simulink model "model"  (R2020b)
settings: Solver=VariableStepAuto  StartTime=0.0  StopTime=settings.Tsim  FixedStep=0.1  RelTol=1e-6  AbsTol=1e-6
values from neighbouring files (symbols this model uses):
  D = date(3)    [date2jd.m]
  settings = Simulink.Parameter    [main.m]
libraries: vrlib x10
(part 2 of 2)

== matlab function model/disturbanceTorques ==
  data: J input; M_disturbance output; r_CG input; A_BN input; A_BL input; S_B input; rr input; vv input; C_D input; rho input; t input; b_B output
function [M_disturbance, b_B] = disturbanceTorquesa(J, r_CG, A_BN, A_BL, S_B, rr, vv, C_D, rho, t)



G = 6.67408e-11;
m_E = 5.972e+24;
kep = car2par(rr, vv, 398600);
a = kep(1); e = kep(2); i = kep(3);
OM = kep(4); om = kep(5); th = kep(6);
R_equat = 6371e+3; % [m]
p = a*(1-e^2);
R = p / (1+e*cos(th)) * 1e+3; % [m]





% Moments of Inertia [kg*m^2]
% (12U Cubesat)
J1 = J(1,1);
J2 = J(2,2);
J3 = J(3,3);





C1 = (J2-J3)/J1;
C2 = (J3-J1)/J2;
C3 = (J1-J2)/J3;






%% Gravity Gradient Torque
c = A_BL * [1;0;0];



M_GG = [- 3*G*m_E/R^3 *C1* c(3)*c(2);
- 3*G*m_E/R^3 *C2* c(1)*c(3);
- 3*G*m_E/R^3 *C3* c(2)*c(1)];



%% SRP Torque @ 600 Km (Direct Solar Rad. + Sun Rad. Reflected by Earth + Earth Rad.)
F_e = 1358 + 580 + 143.4; % [W/m^2]
P = F_e / (3*1e+8);



N_body = 6; % # main body surfaces
N_SP = 4; % # solar panel surfaces



U = 0.1; % 1U length



N = zeros(N_body+N_SP,3);
A = zeros(N_body+N_SP,1);
r = zeros(N_body+N_SP,3);
n1 = [1 0 0]; n2 = [0 1 0]; n3 = [0 0 1];
% S/C Main Body: Normals, Surface Coefficients, Areas
N(1,:) = n1; N(2,:) = n2; N(3,:) = n3;
N(4,:) = -n1; N(5,:) = -n2; N(6,:) = -n3;
rho_s_body = 0.6; rho_d_body = 0.1;
A(1:N_body) = [4 6 6 4 6 6]*U^2; % [m^2]



% Solar Panels: Normals, Surface Coefficients, Areas
N(7,:) = n1; N(8,:) = -n1; N(9,:) = n1; N(10,:) = -n1;
rho_s_SP = 0.6; rho_d_SP = 0.1;
A(N_body+1:N_body+N_SP) = [12 12 12 12]*U^2; % [m^2]



% L.u.c. a RF centered @ Geometric Center of S/C::
% we will use it to define the coordinates of each surface's center
% along w/ the coordinates of th CG w.r.t. GC
r(1,:) = [1.5 0 0]*U; r(2,:) = [0 1 0]*U; r(3,:) = [0 0 1]*U;
r(4,:) = [-1.5 0 0]*U; r(5,:) = [0 -1 0]*U; r(6,:) = [0 0 -1]*U;
r(7,:) = [0 5 0]*U; r(8,:) = [0 5 0]*U;
r(9,:) = [0 -5 0]*U; r(10,:) = [0 -5 0]*U;



S_B_norm = S_B / norm(S_B);



M_SRP = zeros(3,1);
for k = 1:N_body+N_SP
if k <= N_body
rho_s = rho_s_body; rho_d = rho_d_body;
else
rho_s = rho_s_SP; rho_d = rho_d_SP;
end



n_k = N(k,:)';
F_k = - P*A(k)*dot(S_B_norm,n_k) * ( (1-rho_s)*S_B_norm + (2*rho_s*dot(S_B_norm,n_k)+2/3*rho_d)*n_k );



if dot(S_B_norm, n_k) > 0
r_k = (r(k,:) - r_CG')';
M_SRP_k = cross(r_k, F_k);
else
M_SRP_k = zeros(3,1);
end



M_SRP = M_SRP + M_SRP_k;



end




%% Air-Drag Torque
w_E = 2*pi/(23*3600 + 56*60 + 4.09); % Earth's angular rate [rad/s]
mu_E = 398600.433; % [km^3/s^2]



% Rotation matrices: Earth-Centered Inertial --> Perifocal (ECI->PF)
R_om = [cos(om) sin(om) 0 ;
-sin(om) cos(om) 0 ;
0 0 1 ];



R_i = [ 1 0 0 ;
0 cos(i) sin(i);
0 -sin(i) cos(i)];



R_OM = [cos(OM) sin(OM) 0 ;
-sin(OM) cos(OM) 0 ;
0 0 1 ];



R313 = R_om * R_i * R_OM; % ECI --> PF



R_PF = R * [cos(th), sin(th), 0]';
v_PF = sqrt(mu_E/p) * [-sin(th), (e+cos(th)), 0]';
% PF --> ECI
r_ECI = R313'* R_PF;
v_ECI = R313'* v_PF;



v_rel_N = v_ECI + cross([0 0 w_E]', r_ECI);
v_rel_B = A_BN*v_rel_N; % Relative atmosphere velocity (@body frame)
v_rel_B_unit = v_rel_B / norm(v_rel_B);



M_drag = zeros(3,1);
for k = 1:N_body+N_SP



n_k = N(k,:)';
F_k = - .5 * C_D * rho * norm(v_rel_B)^2 * dot(n_k,v_rel_B_unit) * A(k) * v_rel_B_unit;



if dot(S_B_norm, n_k) > 0
r_k = (r(k,:) - r_CG')';
M_drag_k = cross(r_k, F_k);
else
M_drag_k = zeros(3,1);
end



M_drag = M_drag + M_drag_k;



end



%% Magnetic Torque
g10 = -29615e-9; g11 = -1728e-9; h11 = 5186e-9;
H0 = sqrt(g10^2 + g11^2 + h11^2);
m = [sind(11.5)*cos(w_E*t);
sind(11.5)*sin(w_E*t);
cosd(11.5)];
r_N = R * [cos(th);
sin(th)*cos(i);
sin(th)*sin(i)];



% Magnetic field vector
b_N = R_equat^3*H0/R^3 * (3*dot(m/norm(m),r_N/norm(r_N))*r_N/norm(r_N) - m/norm(m));
b_B = A_BN * b_N;
% Parasitic magnetic torque



M_magn = cross(m, b_B);
M_disturbance = [M_drag(:), M_SRP(:), M_magn(:), M_GG(:)];

== matlab function model/SENSORS/Gyroscope/MATLAB Function ==
  data: x input; x_dot output; om input; M output
function [x_dot,M] = GyroModel(x,om)
%gyro inertia parameters
Ir = 1e-7;
Jz = 2e-7;
%tuning parameter for visco-elastic reaction torque
k=10;
%tuning law for c for fastest convergence
c_gyro = 2*sqrt(k*Jz);
om_x = om(1);
om_y = om(2);
om_z = om(3);
%angular velocity of gyro wheel (100 deg/s)
om_r = 100*pi/180;



% defining the theta_i and \dot theta_i
x_dot = zeros(6,1);



th_x = x(1);
th_y = x(2);
th_z = x(3);
va_x = x(4);
va_y = x(5);
va_z = x(6);
%3 gyro dynamics expressed as 1st order differential equation
x_dot(1) = va_x;
x_dot(2) = va_y;
x_dot(3) = va_z;
x_dot(4) = -(c_gyro/Jz)*va_x-(k/Jz)*th_x-(Ir/Jz)*om_r*om_x;
x_dot(5) = -(c_gyro/Jz)*va_y-(k/Jz)*th_y-(Ir/Jz)*om_r*om_y;
x_dot(6) = -(c_gyro/Jz)*va_z-(k/Jz)*th_z-(Ir/Jz)*om_r*om_z;
%gyro outputs
x_dot=[x_dot(1) x_dot(2) x_dot(3) x_dot(4) x_dot(5) x_dot(6)]';



%feedback torque applied to the gyros
M_x = -k*th_x-c_gyro*va_x;
M_y = -k*th_y-c_gyro*va_y;
M_z = -k*th_z-c_gyro*va_z;



M = [M_x M_y M_z]';




end

== matlab function model/SENSORS/Gyroscope/MATLAB Function1 ==
  data: state_vector input; omega_raw output
function omega_raw = fcn(state_vector)



theta_vec = state_vector(1:3);
Ir = 1e-7;
k = 10;
om_r = 100*pi/180;



omega_raw = - k*theta_vec / (Ir*om_r);



end

== matlab function model/CONTROL AND ACTUATORS/RW Moment1 ==
  data: M_onlyMagnetorquer input; M_magnetorquer input; Mc output; M_RW input; tMaxOnlyMagn input; tMaxDetumbling input; t input
function Mc = fcn(M_onlyMagnetorquer, M_magnetorquer, M_RW, tMaxOnlyMagn, tMaxDetumbling, t)

if t <= tMaxOnlyMagn
    Mc = M_onlyMagnetorquer;
elseif t > tMaxOnlyMagn && t <= tMaxDetumbling
    Mc = M_magnetorquer + M_RW;
else
    Mc = M_RW;
end

== matlab function model/CONTROL AND ACTUATORS/MATLAB Function2 ==
  data: MagMax input; B_sensed input; Mc input; D output; M_eff_sensed output
function [D, M_eff_sensed] = fcn(MagMax,B_sensed,Mc)
D=1/dot(B_sensed,B_sensed)*cross(B_sensed,Mc);
if D(1)>MagMax
    D(1)=MagMax;
end
if D(2)>MagMax
    D(2)=MagMax;
end
if D(3)>MagMax
    D(3)=MagMax;
end
M_eff_sensed=cross(D,B_sensed);

== matlab function model/CONTROL AND ACTUATORS/If Action Subsystem2/Target Pointing Algorithm ==
  data: w_b_sensed input; A_e input; Mc output; w_req input; Kp input; Kd input
function Mc  = fcn(w_b_sensed,A_e,w_req,Kp,Kd)

Mx = -Kp(1,1)/2*(A_e(2,3)-A_e(3,2))-Kd(1,1)*(w_b_sensed(1)-w_req(1));
My = -Kp(2,1)/2*(A_e(3,1)-A_e(1,3))-Kd(2,1)*(w_b_sensed(2)-w_req(2));
Mz = -Kp(3,1)/2*(A_e(1,2)-A_e(2,1))-Kd(3,1)*(w_b_sensed(3)-w_req(3));

Mc = [Mx;My;Mz];
